simulink model "ASMC_without_Sensor_Noise"  (R2023a)
settings: Solver=FixedStepAuto  StartTime=0.0  StopTime=30  FixedStep=0.1  RelTol=1e-3
settings Model: Creator=suhas  LastModifiedBy=suhas

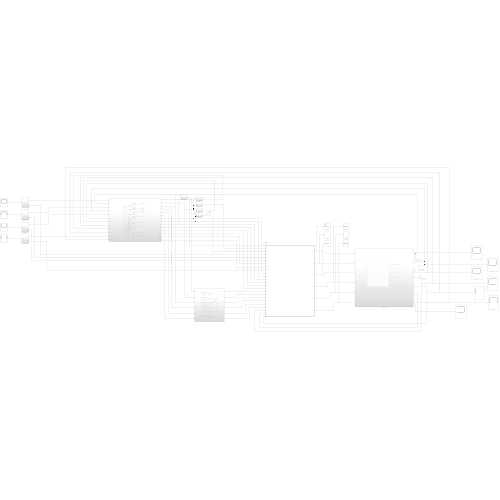
[thumbnail: Simulink's stored preview of the top-level diagram]
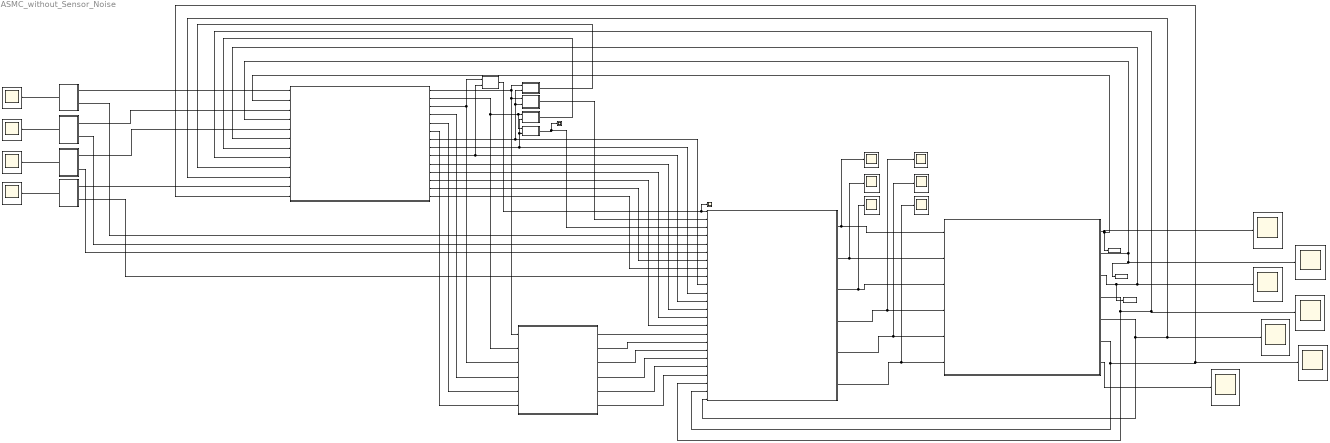
== system ASMC_without_Sensor_Noise ==
  Adaptive Sliding Mode controller : MATLAB Function  TreatAsAtomicUnit=on
  Error Dynamics PSI : Subsystem
      settings: PortSchema="{\"entries\":[{\"content\":{\"sides\":[{\"content\":{\"connectorIds\":[\"Out3\"]},\"type\":\"ConnectorPlacement.EquallySpacedRectSide\",\"uuid\":\"6ff76342-8998-4651-836f-b3548aab8e65\"},{\"content\":{\"connectorIds\":[\"Out1\",\"Out2\"],\"side\":\"RIGHT\"},\"type\":\"ConnectorPlacement.EquallySpacedRectSide\",\"uuid\":\"ba3c50f9-7a2f-41a1-a732-e8b3bac2c00e\"},{\"content\":{\"side\":\"TOP\"},\"type\":\"ConnectorPlacement.EquallySpacedRectSide\",\"uuid\":\"514097a0-d1ba-49fb-95f6-b3a102a24ffc\"}]},\"type\":\"ConnectorPlacement.EquallySpacedConnector\",\"uuid\":\"1840ab09-275d-484b-96f5-5e7a2fe55b85\"}],\"packageUris\":[\"http://schema.mathworks.com/mf0/Connector/R2020b\"],\"version\":\"1.0\"}"
  Error Dynamics X : Subsystem
      settings: PortSchema="{\"entries\":[{\"content\":{\"sides\":[{\"content\":{\"connectorIds\":[\"Out3\"]},\"type\":\"ConnectorPlacement.EquallySpacedRectSide\",\"uuid\":\"22545104-e9c6-42c1-9867-858d35d84d65\"},{\"content\":{\"connectorIds\":[\"Out1\",\"Out2\"],\"side\":\"RIGHT\"},\"type\":\"ConnectorPlacement.EquallySpacedRectSide\",\"uuid\":\"13e23cfd-25ed-4968-b510-5096e9888b79\"},{\"content\":{\"side\":\"TOP\"},\"type\":\"ConnectorPlacement.EquallySpacedRectSide\",\"uuid\":\"a5842cd3-47ad-4199-b3b5-f0c05b0cfae5\"}]},\"type\":\"ConnectorPlacement.EquallySpacedConnector\",\"uuid\":\"431437ec-b026-4082-bc82-4a08cacc56be\"}],\"packageUris\":[\"http://schema.mathworks.com/mf0/Connector/R2020b\"],\"version\":\"1.0\"}"
  Error Dynamics Y : Subsystem
      settings: PortSchema="{\"entries\":[{\"content\":{\"sides\":[{\"content\":{\"connectorIds\":[\"Out3\"]},\"type\":\"ConnectorPlacement.EquallySpacedRectSide\",\"uuid\":\"22545104-e9c6-42c1-9867-858d35d84d65\"},{\"content\":{\"connectorIds\":[\"Out1\",\"Out2\"],\"side\":\"RIGHT\"},\"type\":\"ConnectorPlacement.EquallySpacedRectSide\",\"uuid\":\"13e23cfd-25ed-4968-b510-5096e9888b79\"},{\"content\":{\"side\":\"TOP\"},\"type\":\"ConnectorPlacement.EquallySpacedRectSide\",\"uuid\":\"a5842cd3-47ad-4199-b3b5-f0c05b0cfae5\"}]},\"type\":\"ConnectorPlacement.EquallySpacedConnector\",\"uuid\":\"431437ec-b026-4082-bc82-4a08cacc56be\"}],\"packageUris\":[\"http://schema.mathworks.com/mf0/Connector/R2020b\"],\"version\":\"1.0\"}"
  Error Dynamics Z : Subsystem
      settings: PortSchema="{\"entries\":[{\"content\":{\"sides\":[{\"content\":{\"connectorIds\":[\"Out3\"]},\"type\":\"ConnectorPlacement.EquallySpacedRectSide\",\"uuid\":\"6ff76342-8998-4651-836f-b3548aab8e65\"},{\"content\":{\"connectorIds\":[\"Out1\",\"Out2\"],\"side\":\"RIGHT\"},\"type\":\"ConnectorPlacement.EquallySpacedRectSide\",\"uuid\":\"ba3c50f9-7a2f-41a1-a732-e8b3bac2c00e\"},{\"content\":{\"side\":\"TOP\"},\"type\":\"ConnectorPlacement.EquallySpacedRectSide\",\"uuid\":\"514097a0-d1ba-49fb-95f6-b3a102a24ffc\"}]},\"type\":\"ConnectorPlacement.EquallySpacedConnector\",\"uuid\":\"1840ab09-275d-484b-96f5-5e7a2fe55b85\"}],\"packageUris\":[\"http://schema.mathworks.com/mf0/Connector/R2020b\"],\"version\":\"1.0\"}"
  Error Generator : Subsystem
  Estimated  ground effect : Subsystem
  Estimated Input u5 (v6) : Subsystem
  Estimated Input u6 (v6) : Subsystem
  Phi Estimated : Subsystem
  Phi Scope : Scope
  Psi Scope : Scope
  Quadcopter Dynamics : Subsystem
  Scope{,1..2,4..6} (6 alike) : Scope
  Sliding Surface (S) : Subsystem
  Theta Desired : Subsystem
  Theta Scope : Scope
  To Workspace : ToWorkspace  VariableName=x  SaveFormat=Timeseries  SampleTime=-1
  To Workspace1 : ToWorkspace  VariableName=y  SaveFormat=Timeseries  SampleTime=-1
  To Workspace2 : ToWorkspace  VariableName=z  SaveFormat=Timeseries  SampleTime=-1
  X Scope : Scope
  Y Scope : Scope
  Z Scope : Scope
  gr scope : Scope
  u1 Scope : Scope
  u2 Scope : Scope
  u3 Scope : Scope
  u4 Scope : Scope
  u5 Scope : Scope
  u6 Scope : Scope
  wires:
  Quadcopter Dynamics/6(psi) -> Adaptive Sliding Mode controller/23(psi), Error Generator/12(psi), Psi Scope/1
  Adaptive Sliding Mode controller/1(u1) -> Quadcopter Dynamics/1(u1), u1 Scope/1
  Error Dynamics Y/2(yd_ddot) -> Adaptive Sliding Mode controller/5(yd_dd)
  Error Dynamics PSI/2(psid_ddot) -> Adaptive Sliding Mode controller/9(psid_dd)
  Error Dynamics Z/1(zd) -> Error Generator/5(zd)
  Sliding Surface (S)/5(s5) -> Adaptive Sliding Mode controller/20(s5)
  Quadcopter Dynamics/5(theta) -> Adaptive Sliding Mode controller/24(theta), Theta Scope/1, Error Generator/10(theta)
  Sliding Surface (S)/4(s4) -> Adaptive Sliding Mode controller/19(s4)
  Error Dynamics PSI/1(psid) -> Error Generator/11(psid)
  Error Generator/5(etheta) -> Sliding Surface (S)/5(thetae)
  Error Generator/2(ey) -> Estimated Input u6 (v6)/1(ey), Phi Estimated/1(ey), Sliding Surface (S)/2(ye)
  Error Generator/4(ephi) -> Sliding Surface (S)/4(phie)
  Error Generator/10(ephid) -> Adaptive Sliding Mode controller/13(ephid)
  Error Generator/7(exd) -> Adaptive Sliding Mode controller/10(exd), Estimated Input u5 (v6)/2(exd), Theta Desired/2(exd)
  Adaptive Sliding Mode controller/5(u5) -> Quadcopter Dynamics/5(u5), u5 Scope/1
  Error Generator/13(phid_dd) -> Adaptive Sliding Mode controller/7(phid_dd)
  Adaptive Sliding Mode controller/6(u6) -> Quadcopter Dynamics/6(u6), u6 Scope/1
  Quadcopter Dynamics/4(phi) -> Adaptive Sliding Mode controller/22(phi), Phi Scope/1, Error Generator/8(phi)
  Error Dynamics Y/1(yd) -> Error Generator/3(yd)
  Error Generator/9(ezd) -> Estimated  ground effect/2(ezd), Adaptive Sliding Mode controller/12(ezd)
  Error Generator/6(epsi) -> Sliding Surface (S)/6(psie)
  Adaptive Sliding Mode controller/3(u3) -> u3 Scope/1, Quadcopter Dynamics/3(u3)
  Quadcopter Dynamics/3(z) -> Z Scope/1, Error Generator/6(z), To Workspace2/1
  Error Generator/8(eyd) -> Adaptive Sliding Mode controller/11(eyd), Phi Estimated/2(eyd), Estimated Input u6 (v6)/2(eyd)
  Error Generator/12(epsid) -> Adaptive Sliding Mode controller/15(epsid)
  Error Dynamics X/2(xd_ddot) -> Adaptive Sliding Mode controller/4(xd_dd)
  Adaptive Sliding Mode controller/4(u4) -> Quadcopter Dynamics/4(u4), u4 Scope/1
  Sliding Surface (S)/1(s1) -> Adaptive Sliding Mode controller/16(s1)
  Error Generator/14(thetad_dd) -> Adaptive Sliding Mode controller/8(thetad_dd)
  Error Generator/11(ethetad) -> Adaptive Sliding Mode controller/14(ethetad)
  Error Generator/3(ez) -> Estimated  ground effect/1(ez), Sliding Surface (S)/3(ze)
  Quadcopter Dynamics/1(x) -> Error Generator/2(x), To Workspace/1, X Scope/1
  Adaptive Sliding Mode controller/2(u2) -> Quadcopter Dynamics/2(u2), u2 Scope/1
  Sliding Surface (S)/2(s2) -> Adaptive Sliding Mode controller/17(s2)
  Quadcopter Dynamics/2(y) -> Y Scope/1, To Workspace1/1, Error Generator/4(y)
  Sliding Surface (S)/3(s3) -> Adaptive Sliding Mode controller/18(s3)
  Error Dynamics Z/2(zd_ddot) -> Adaptive Sliding Mode controller/6(zd_dd)
  Error Dynamics X/1(xd) -> Error Generator/1(xd)
  Sliding Surface (S)/6(s6) -> Adaptive Sliding Mode controller/21(s6)
  Error Generator/1(ex) -> Sliding Surface (S)/1(xe), Estimated Input u5 (v6)/1(ex), Theta Desired/1(ex)
  Estimated Input u5 (v6)/1(v5) -> Adaptive Sliding Mode controller/2(v5)
  Estimated Input u6 (v6)/1(v6) -> Scope5/1, Adaptive Sliding Mode controller/3(v6)
  Estimated  ground effect/1(fr) -> Scope6/1, Adaptive Sliding Mode controller/1(fr)
  Theta Desired/1(thetad) -> Error Generator/9(thetad)
  Phi Estimated/1(phid) -> Error Generator/7(phid)
  Error Dynamics X/3(x) -> Scope/1
  Error Dynamics Y/3(y) -> Scope1/1
  Error Dynamics Z/3(z) -> Scope2/1
  Error Dynamics PSI/3(psi) -> Scope4/1
  Quadcopter Dynamics/7(gr) -> gr scope/1

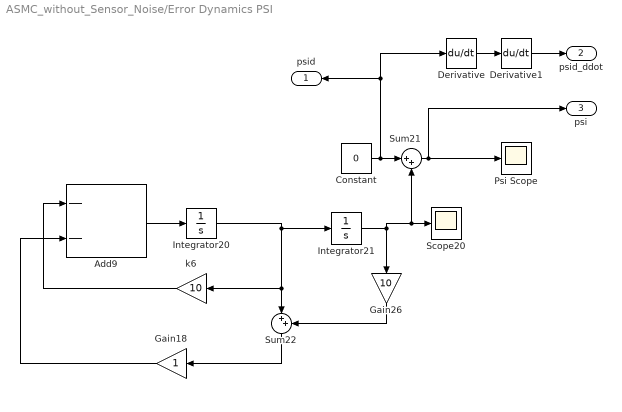
== system ASMC_without_Sensor_Noise/Error Dynamics PSI ==
  Add9 : Sum  Inputs=--
  Constant : Constant  Value=0
  Derivative : Derivative
  Derivative1 : Derivative
  Gain18 : Gain
  Gain26 : Gain  Gain=10
  Integrator20 : Integrator
  Integrator21 : Integrator  InitialCondition=0.5235
  Psi Scope : Scope
  Scope20 : Scope
  Sum21 : Sum  Inputs=|++
  Sum22 : Sum  Inputs=|++
  k6 : Gain  Gain=10
  psid : Outport
  psid_ddot : Outport  Port=2
  psi : Outport  Port=3
  wires:
  Integrator20/1 -> Integrator21/1, k6/1, Sum22/1
  k6/1 -> Add9/1
  Sum21/1 -> psi/1, Psi Scope/1
  Add9/1 -> Integrator20/1
  Gain26/1 -> Sum22/2
  Gain18/1 -> Add9/2
  Integrator21/1 -> Sum21/2, Scope20/1, Gain26/1
  Sum22/1 -> Gain18/1
  Constant/1 -> psid/1, Derivative/1, Sum21/1
  Derivative/1 -> Derivative1/1
  Derivative1/1 -> psid_ddot/1

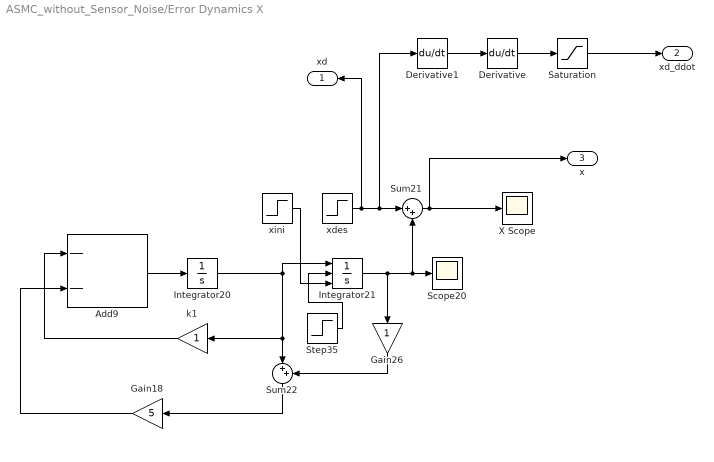
== system ASMC_without_Sensor_Noise/Error Dynamics X ==
  Add9 : Sum  Inputs=--
  Derivative : Derivative
  Derivative1 : Derivative
  Gain18 : Gain  Gain=5
  Gain26 : Gain
  Integrator20 : Integrator
  Integrator21 : Integrator  ExternalReset=rising  InitialConditionSource=external
  Saturation : Saturate  UpperLimit=100  LowerLimit=-100
  Scope20 : Scope
  Step35 : Step  Time=15  SampleTime=0
  Sum21 : Sum  Inputs=|++
  Sum22 : Sum  Inputs=|++
  X Scope : Scope
  k1 : Gain
  xdes : Step  Time=15  Before=20  After=0  SampleTime=0
  xini : Step  Time=15  Before=-10  After=20  SampleTime=0
  xd : Outport
  xd_ddot : Outport  Port=2
  x : Outport  Port=3
  wires:
  Integrator20/1 -> Integrator21/1, k1/1, Sum22/1
  k1/1 -> Add9/1
  Step35/1 -> Integrator21/2
  xdes/1 -> xd/1, Derivative1/1, Sum21/1
  xini/1 -> Integrator21/3
  Sum21/1 -> x/1, X Scope/1
  Add9/1 -> Integrator20/1
  Gain26/1 -> Sum22/2
  Gain18/1 -> Add9/2
  Integrator21/1 -> Gain26/1, Sum21/2, Scope20/1
  Sum22/1 -> Gain18/1
  Derivative1/1 -> Derivative/1
  Derivative/1 -> Saturation/1
  Saturation/1 -> xd_ddot/1

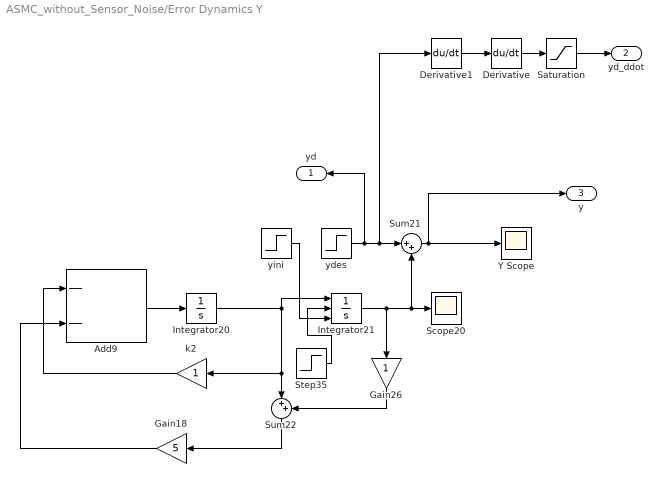
== system ASMC_without_Sensor_Noise/Error Dynamics Y ==
  Add9 : Sum  Inputs=--
  Derivative : Derivative
  Derivative1 : Derivative
  Gain18 : Gain  Gain=5
  Gain26 : Gain
  Integrator20 : Integrator
  Integrator21 : Integrator  ExternalReset=rising  InitialConditionSource=external
  Saturation : Saturate  UpperLimit=100  LowerLimit=-100
  Scope20 : Scope
  Step35 : Step  Time=15  SampleTime=0
  Sum21 : Sum  Inputs=|++
  Sum22 : Sum  Inputs=|++
  Y Scope : Scope
  k2 : Gain
  ydes : Step  Time=15  Before=-10  After=0  SampleTime=0
  yini : Step  Time=15  Before=20  After=-10  SampleTime=0
  yd : Outport
  yd_ddot : Outport  Port=2
  y : Outport  Port=3
  wires:
  Integrator20/1 -> Integrator21/1, k2/1, Sum22/1
  k2/1 -> Add9/1
  Step35/1 -> Integrator21/2
  ydes/1 -> yd/1, Derivative1/1, Sum21/1
  yini/1 -> Integrator21/3
  Sum21/1 -> y/1, Y Scope/1
  Add9/1 -> Integrator20/1
  Gain26/1 -> Sum22/2
  Gain18/1 -> Add9/2
  Integrator21/1 -> Gain26/1, Sum21/2, Scope20/1
  Sum22/1 -> Gain18/1
  Derivative1/1 -> Derivative/1
  Derivative/1 -> Saturation/1
  Saturation/1 -> yd_ddot/1

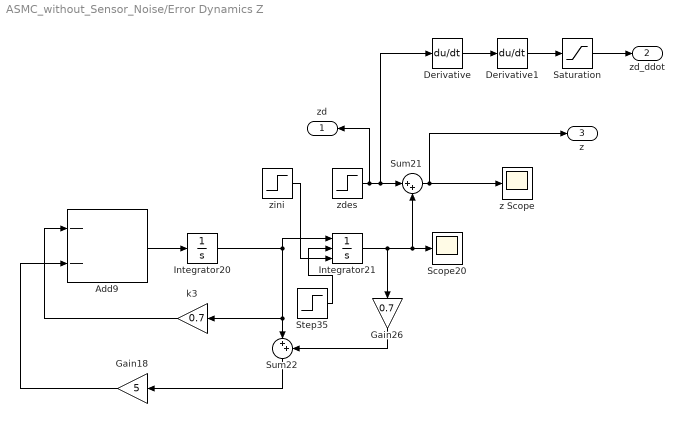
== system ASMC_without_Sensor_Noise/Error Dynamics Z ==
  Add9 : Sum  Inputs=--
  Derivative : Derivative
  Derivative1 : Derivative
  Gain18 : Gain  Gain=5
  Gain26 : Gain  Gain=0.7
  Integrator20 : Integrator
  Integrator21 : Integrator  ExternalReset=rising  InitialConditionSource=external
  Saturation : Saturate  UpperLimit=100  LowerLimit=-100
  Scope20 : Scope
  Step35 : Step  Time=15  SampleTime=0
  Sum21 : Sum  Inputs=|++
  Sum22 : Sum  Inputs=|++
  k3 : Gain  Gain=0.7
  z Scope : Scope
  zdes : Step  Time=15  Before=10  After=0  SampleTime=0
  zini : Step  Time=15  Before=10  After=010  SampleTime=0
  zd : Outport
  zd_ddot : Outport  Port=2
  z : Outport  Port=3
  wires:
  Integrator20/1 -> Integrator21/1, k3/1, Sum22/1
  k3/1 -> Add9/1
  Step35/1 -> Integrator21/2
  zdes/1 -> zd/1, Derivative/1, Sum21/1
  zini/1 -> Integrator21/3
  Sum21/1 -> z/1, z Scope/1
  Add9/1 -> Integrator20/1
  Gain26/1 -> Sum22/2
  Gain18/1 -> Add9/2
  Integrator21/1 -> Gain26/1, Sum21/2, Scope20/1
  Sum22/1 -> Gain18/1
  Derivative/1 -> Derivative1/1
  Derivative1/1 -> Saturation/1
  Saturation/1 -> zd_ddot/1

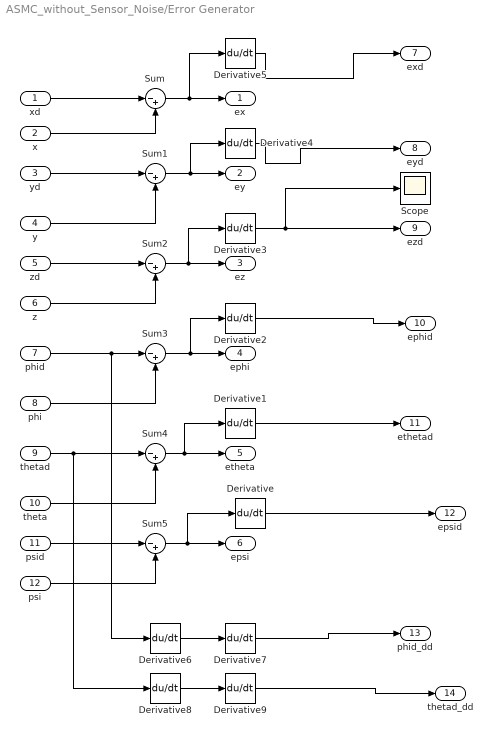
== system ASMC_without_Sensor_Noise/Error Generator ==
  xd : Inport
  x : Inport  Port=2
  yd : Inport  Port=3
  y : Inport  Port=4
  zd : Inport  Port=5
  z : Inport  Port=6
  phid : Inport  Port=7
  phi : Inport  Port=8
  thetad : Inport  Port=9
  theta : Inport  Port=10
  psid : Inport  Port=11
  psi : Inport  Port=12
  Derivative{,1..9} (10 alike) : Derivative
  Scope : Scope
  Sum{,1..5} (6 alike) : Sum  Inputs=|-+
  ex : Outport
  ey : Outport  Port=2
  ez : Outport  Port=3
  ephi : Outport  Port=4
  etheta : Outport  Port=5
  epsi : Outport  Port=6
  exd : Outport  Port=7
  eyd : Outport  Port=8
  ezd : Outport  Port=9
  ephid : Outport  Port=10
  ethetad : Outport  Port=11
  epsid : Outport  Port=12
  phid_dd : Outport  Port=13
  thetad_dd : Outport  Port=14
  wires:
  xd/1 -> Sum/1
  x/1 -> Sum/2
  yd/1 -> Sum1/1
  y/1 -> Sum1/2
  zd/1 -> Sum2/1
  z/1 -> Sum2/2
  phid/1 -> Derivative6/1, Sum3/1
  phi/1 -> Sum3/2
  thetad/1 -> Derivative8/1, Sum4/1
  theta/1 -> Sum4/2
  psid/1 -> Sum5/1
  psi/1 -> Sum5/2
  Sum/1 -> Derivative5/1, ex/1
  Sum1/1 -> Derivative4/1, ey/1
  Sum2/1 -> Derivative3/1, ez/1
  Sum3/1 -> Derivative2/1, ephi/1
  Sum4/1 -> Derivative1/1, etheta/1
  Sum5/1 -> Derivative/1, epsi/1
  Derivative6/1 -> Derivative7/1
  Derivative8/1 -> Derivative9/1
  Derivative3/1 -> ezd/1, Scope/1
  Derivative4/1 -> eyd/1
  Derivative5/1 -> exd/1
  Derivative/1 -> epsid/1
  Derivative7/1 -> phid_dd/1
  Derivative9/1 -> thetad_dd/1
  Derivative1/1 -> ethetad/1
  Derivative2/1 -> ephid/1

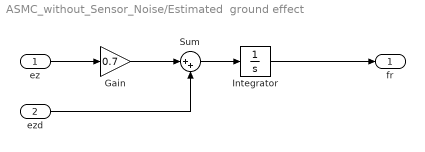
== system ASMC_without_Sensor_Noise/Estimated  ground effect ==
  ez : Inport
  ezd : Inport  Port=2
  Gain : Gain  Gain=0.7
  Integrator : Integrator
  Sum : Sum  Inputs=|++
  fr : Outport
  wires:
  ezd/1 -> Sum/2
  ez/1 -> Gain/1
  Gain/1 -> Sum/1
  Sum/1 -> Integrator/1
  Integrator/1 -> fr/1

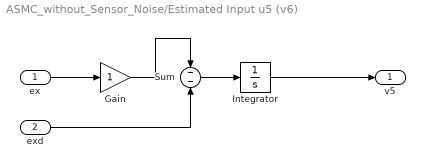
== system ASMC_without_Sensor_Noise/Estimated Input u5 (v6) ==
  ex : Inport
  exd : Inport  Port=2
  Gain : Gain
  Integrator : Integrator
  Sum : Sum  Inputs=--
  v5 : Outport
  wires:
  exd/1 -> Sum/2
  ex/1 -> Gain/1
  Gain/1 -> Sum/1
  Sum/1 -> Integrator/1
  Integrator/1 -> v5/1

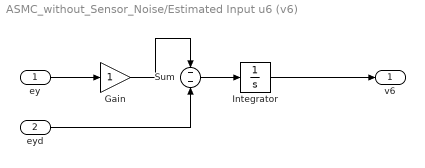
== system ASMC_without_Sensor_Noise/Estimated Input u6 (v6) ==
  ey : Inport
  eyd : Inport  Port=2
  Gain : Gain
  Integrator : Integrator
  Sum : Sum  Inputs=--
  v6 : Outport
  wires:
  eyd/1 -> Sum/2
  ey/1 -> Gain/1
  Gain/1 -> Sum/1
  Sum/1 -> Integrator/1
  Integrator/1 -> v6/1

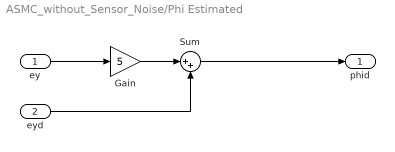
== system ASMC_without_Sensor_Noise/Phi Estimated ==
  ey : Inport
  eyd : Inport  Port=2
  Gain : Gain  Gain=5
  Sum : Sum  Inputs=|++
  phid : Outport
  wires:
  ey/1 -> Gain/1
  Gain/1 -> Sum/1
  Sum/1 -> phid/1
  eyd/1 -> Sum/2

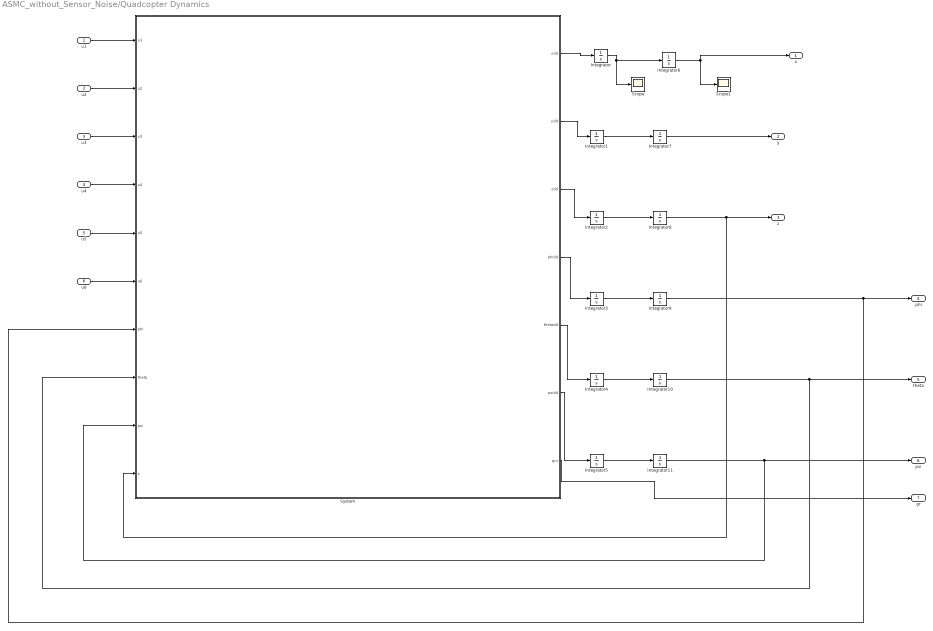
== system ASMC_without_Sensor_Noise/Quadcopter Dynamics ==
  u1 : Inport
  u2 : Inport  Port=2
  u3 : Inport  Port=3
  u4 : Inport  Port=4
  u5 : Inport  Port=5
  u6 : Inport  Port=6
  Integrator : Integrator  UpperSaturationLimit=10  LowerSaturationLimit=-10
  Integrator{1..5} (5 alike) : Integrator
  Integrator10 : Integrator  InitialCondition=0.5235  UpperSaturationLimit=3.14  LowerSaturationLimit=-3.14  WrapState=on
  Integrator11 : Integrator  InitialCondition=0.5235
  Integrator6 : Integrator  InitialCondition=10  UpperSaturationLimit=10  LowerSaturationLimit=0
  Integrator7 : Integrator  InitialCondition=10
  Integrator8 : Integrator  InitialCondition=20
  Integrator9 : Integrator  InitialCondition=0.5235  UpperSaturationLimit=3.14  LowerSaturationLimit=-3.14  WrapState=on  WrappedStateUpperValue=pi/2  WrappedStateLowerValue=-pi/2
  Scope : Scope
  Scope1 : Scope
  System : MATLAB Function  TreatAsAtomicUnit=on
  x : Outport
  y : Outport  Port=2
  z : Outport  Port=3
  phi : Outport  Port=4
  theta : Outport  Port=5
  psi : Outport  Port=6
  gr : Outport  Port=7
  wires:
  u1/1 -> System/1(u1)
  u2/1 -> System/2(u2)
  u3/1 -> System/3(u3)
  u4/1 -> System/4(u4)
  u5/1 -> System/5(u5)
  u6/1 -> System/6(u6)
  System/1(xdd) -> Integrator/1
  System/2(ydd) -> Integrator1/1
  System/3(zdd) -> Integrator2/1
  System/4(phidd) -> Integrator3/1
  System/5(thetadd) -> Integrator4/1
  System/6(psidd) -> Integrator5/1
  Integrator1/1 -> Integrator7/1
  Integrator2/1 -> Integrator8/1
  Integrator3/1 -> Integrator9/1
  Integrator4/1 -> Integrator10/1
  Integrator5/1 -> Integrator11/1
  Integrator10/1 -> theta/1, System/8(theta)
  Integrator11/1 -> psi/1, System/9(psi)
  Integrator9/1 -> phi/1, System/7(phi)
  Integrator8/1 -> z/1, System/10(z)
  Integrator7/1 -> y/1
  Integrator6/1 -> x/1, Scope1/1
  Integrator/1 -> Integrator6/1, Scope/1
  System/7(grz) -> gr/1

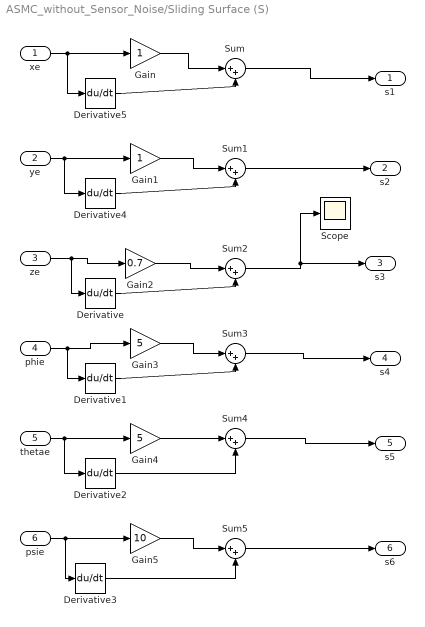
== system ASMC_without_Sensor_Noise/Sliding Surface (S) ==
  xe : Inport
  ye : Inport  Port=2
  ze : Inport  Port=3
  phie : Inport  Port=4
  thetae : Inport  Port=5
  psie : Inport  Port=6
  Derivative{,1..5} (6 alike) : Derivative
  Gain : Gain
  Gain1 : Gain
  Gain2 : Gain  Gain=0.7
  Gain3 : Gain  Gain=5
  Gain4 : Gain  Gain=5
  Gain5 : Gain  Gain=10
  Scope : Scope
  Sum{,1..5} (6 alike) : Sum  Inputs=|++
  s1 : Outport
  s2 : Outport  Port=2
  s3 : Outport  Port=3
  s4 : Outport  Port=4
  s5 : Outport  Port=5
  s6 : Outport  Port=6
  wires:
  xe/1 -> Derivative5/1, Gain/1
  Sum5/1 -> s6/1
  Sum4/1 -> s5/1
  Sum3/1 -> s4/1
  Sum2/1 -> Scope/1, s3/1
  Sum1/1 -> s2/1
  Sum/1 -> s1/1
  Gain/1 -> Sum/1
  Derivative5/1 -> Sum/2
  ye/1 -> Derivative4/1, Gain1/1
  Gain1/1 -> Sum1/1
  Derivative4/1 -> Sum1/2
  ze/1 -> Derivative/1, Gain2/1
  Derivative/1 -> Sum2/2
  Gain2/1 -> Sum2/1
  phie/1 -> Derivative1/1, Gain3/1
  Derivative1/1 -> Sum3/2
  Gain3/1 -> Sum3/1
  thetae/1 -> Derivative2/1, Gain4/1
  Derivative2/1 -> Sum4/2
  Gain4/1 -> Sum4/1
  psie/1 -> Derivative3/1, Gain5/1
  Derivative3/1 -> Sum5/2
  Gain5/1 -> Sum5/1

== system ASMC_without_Sensor_Noise/Theta Desired ==
  ex : Inport
  exd : Inport  Port=2
  Gain : Gain  Gain=5
  Sum : Sum  Inputs=|++
  thetad : Outport
  wires:
  ex/1 -> Gain/1
  Gain/1 -> Sum/1
  Sum/1 -> thetad/1
  exd/1 -> Sum/2

== matlab function ASMC_without_Sensor_Noise/Adaptive Sliding Mode controller ==
  data: fr input; u1 output; v5 input; v6 input; xd_dd input; yd_dd input; zd_dd input; phid_dd input; thetad_dd input; psid_dd input; exd input; eyd input; ezd input; ephid input; ethetad input; epsid input; s1 input; s2 input; s3 input; s4 input; s5 input; s6 input; u2 output; u3 output; u4 output; u5 output; u6 output; phi input; psi input; theta input
function [u1,u2,u3,u4,u5,u6] = fcn(fr,v5,v6,xd_dd,yd_dd,zd_dd,phid_dd,thetad_dd,psid_dd,exd,eyd,ezd,ephid,ethetad,epsid,s1,s2,s3,s4,s5,s6,phi,psi,theta) 

%% G1=[[0,0,0,0,1,0];[0,0,0,0,0,1];[1,0,0,0,0,0];[0,1,0,0,0,0];[0,0,1,0,0,0];[0,0,0,1,0,0]];
G2=[[(cos(phi)*sin(theta)*cos(psi))+(sin(phi)*sin(psi)),0,0,0,1,0];[(cos(phi)*sin(theta)*sin(psi))-(sin(phi)*cos(psi)),0,0,0,0,1];[cos(phi)*cos(theta),0,0,0,0,0];[0,1,0,0,0,0];[0,0,1,0,0,0];[0,0,0,1,0,0]];
F=[0;0;-9.81;0;0;0];
FR=[0;0;fr;0;0;0];
v=[v5;v6;0;0;0;0];
xDdd=[xd_dd;yd_dd;zd_dd;phid_dd;thetad_dd;psid_dd];
ed=[exd;eyd;0.7*ezd;5*ephid;5*ethetad;10*epsid];
cs=[5*s1;5*s2;5*s3;s4;s5;s6];
inner=v-FR-F+xDdd-ed-cs;
final=inv(G2)*inner;
u1=final(1,1);
u2=final(2,1);
u3=final(3,1);
u4=final(4,1);
u5=final(5,1);
u6=final(6,1);

== matlab function ASMC_without_Sensor_Noise/Quadcopter Dynamics/System ==
  data: u1 input; u2 input; u3 input; u4 input; u5 input; u6 input; xdd output; ydd output; zdd output; phidd output; thetadd output; psidd output; phi input; theta input; psi input; z input; grz output
function [xdd,ydd,zdd,phidd,thetadd,psidd,grz] = fcn(u1,u2,u3,u4,u5,u6,phi,theta,psi,z)

%% G1=[[0,0,0,0,1,0];[0,0,0,0,0,1];[1,0,0,0,0,0];[0,1,0,0,0,0];[0,0,1,0,0,0];[0,0,0,1,0,0]];
G2=[[(cos(phi)*sin(theta)*cos(psi))+(sin(phi)*sin(psi)),0,0,0,1,0];[(cos(phi)*sin(theta)*sin(psi))-(sin(phi)*cos(psi)),0,0,0,0,1];[cos(phi)*cos(theta),0,0,0,0,0];[0,1,0,0,0,0];[0,0,1,0,0,0];[0,0,0,1,0,0]];

%% v=[u5;u6;0;0;0;0];
A=0.4668;

if z<2
    grz=A*((1/z^2)-1/4);
else 
    grz=0;
end

fx=[0;0;-9.81;0;0;0];
frx=[0;0;grz;0;0;0];
U=[u1;u2;u3;u4;u5;u6];

%% Xdd=fx+(G*U)-v+frx;
Xdd=fx+(G2*U)+frx;

xdd=Xdd(1,1);
ydd=Xdd(2,1);
zdd=Xdd(3,1);
phidd=Xdd(4,1);
thetadd=Xdd(5,1);
psidd=Xdd(6,1);
